simulink model "twozonevavdemo"  (R2020a)
settings: Solver=FixedStepAuto  StartTime=0  StopTime=24*3600  FixedStep=0.1  RelTol=1e-3
PostLoadFcn:
  | if any(exist('dsrtsu_mdlpostloadfcn', 'file') ~= 0), dsrtsu_mdlpostloadfcn('Execute', bdroot); end
InitFcn:
  | , if any(exist('rtifpga_mdlclblib', 'file') ~= 0), rtifpga_mdlclblib('Init', bdroot); end,
  | , if any(exist('dsmpb_private', 'file') ~= 0), dsmpb_private('dsmpb_mdlclblib', 'Init', bdroot); end,
undefined symbols (not defined in the file): dspaceexample_t_dy975j4bckM, newDymolaGui
libraries: dsmpblib x10
PreSaveFcn:
  | , if any(exist('dsmpb_private', 'file') ~= 0), dsmpb_private('dsmpb_mdlclblib', 'PreSave', bdroot); end,
CloseFcn:
  | , if any(exist('dsmpb_private', 'file') ~= 0), dsmpb_private('dsmpb_mdlclblib', 'Close', bdroot); end,
settings Model: RTICANMMDATA=struct('GeneralSetupData',struct('modelroot','D:\github\dspace-modelica-example\simulink\twozonevavdemo','generalsettings',struct('filesettings',struct('destfolder',struct('Name','RTICANMM_FILES','Check',1),'buildfolder',struct('Name','.','Check',1),'AbsDestfolder',struct('Name','D:\github\dspace-modelica-example\simulink\twozonevavdemo\RTICANMM_FILES'),'AbsBuildfolder',struct('Name','D:\github\dspace-modelica-example\simulink\twozonevavdemo'))),'options',struct('addpaths',1,'rmpaths',1,'addtrcexclusion',true,'cannavigator',struct('checkmonitoring',0),'show_usrtrc',0,'use_usrtrc',0),'advanced',struct('options',ones(1,100)),'MPSetup',{{}},'RTI',struct('Type','DSRT','Ver','4.3','Date','02-May-2020'),'modelname','twozonevavdemo','block','twozonevavdemo'))  DSRTSU_INTERNAL_RTIFPGA=160  DSMPB_ID_DATA={'100',struct('BlockId','6dd11bb4-ebec-4f08-8ba6-7ddbcbec7d3b','SignalIds',{{'2fb2bb90-4ec6-48ad-8f81-f1d196760c71'}}),'101',struct('BlockId','2ef807c6-571a-44f3-9a64-946af00fb830','SignalIds',{{'b929fcdd-48af-480b-af6b-b2c3ef490cf9'}}),'102',struct('BlockId','fcb8ffc9-48d0-43e3-97e6-63db34e8a87a','SignalIds',{{'7405cf0b-34b8-4d18-b681-bf257a32f1fc'}}),'103',struct('BlockId','44e3c1f1-df5a-4dd4-b5d4-1957fbd80a33','SignalIds',{{'7449a4d7-6efa-496e-ad1d-0eb127210326'}}),'104',struct('BlockId','d3fc6cbc-e5ea-45da-a1ff-e6d33e572c72','SignalIds',{{'ae88789f-7deb-4ded-bc5a-6d8a92166d0d'}}),'199',struct('BlockId','9376efae-c5ba-4aee-a189-875ca35da0c2','SignalIds',{{'13f0521d-e993-4fe3-8f8d-d5fdd3bf7eee'}}),'200',struct('BlockId','0e030ddc-3f5d-48b0-903c-79a8b3e79f79','SignalIds',{{'2dba2b15-4113-4beb-a147-18d9996277b5'}}),'97',struct('BlockId','c439f065-e928-4c50-b5e3-14eb295499a2','SignalIds',{{'8fe5f31b-da93-4239-8dda-b4cd2b1e3d5b'}}),'98',struct('BlockId','8b35e11d-29bf-41ba-bcb3-e0861426f11f','SignalIds',{{'ce953cd3-6947-465f-be2f-d959c5a96f49'}}),'99',struct('BlockId','4007e34d-3596-41e8-9571-21578a657730','SignalIds',{{'6190f487-0612-4ce8-bb29-664a6f7d7b4d'}})}  Creator=yangyang.fu  LastModifiedBy=yangyang.fu
settings OptimizationCC: BlockReduction=off  ConditionallyExecuteInputs=off  OptimizeBlockIOStorage=off  BufferReuse=off
settings DebuggingCC: TasksWithSamePriorityMsg=none
settings HardwareCC: ProdBitPerPointer=32  ProdBitPerSizeT=32  ProdBitPerPtrDiffT=32  ProdLargestAtomicInteger=Integer  ProdWordSize=32  ProdLongLongMode=on  ProdHWDeviceType=Custom Processor->Custom
settings ModelReferenceCC: EnableParallelModelReferenceBuilds=on
settings SFSimCC: MATLABDynamicMemAlloc=off
settings RTWCC: Description=dSPACE Run-Time Target (for VEOS on Windows and ConfigurationDesk)  SystemTargetFile=dsrt.tlc  GenCodeOnly=on  MakeCommand=make_dsrt  TemplateMakefile=dsrt_default_tmf  RTWVerbose=off  CustomInclude="\"C:\\Program Files\\Dymola 2021\\Source\""
settings STFCustomTargetCC: TargetLangStandard=C99 (ISO)  ParMdlRefBuildCompliant=on  SystemTargetFile=dsrt.tlc
settings GRTTargetCC: CompOptLevelCompliant=off  ConcurrentExecutionCompliant=off  CombineOutputUpdateFcns=off  MatFileLogging=off  CPPClassGenCompliant=off  UseToolchainInfoCompliant=off

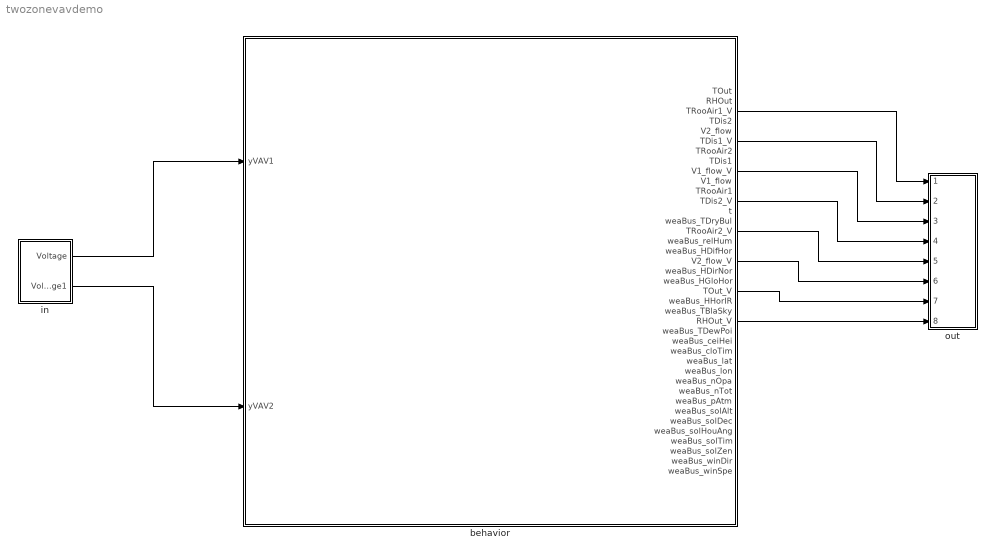
== system twozonevavdemo ==
  behavior : Subsystem
  in : Subsystem
  out : Subsystem
  wires:
  in/1(Voltage) -> behavior/1(yVAV1)
  in/2(Voltage1) -> behavior/2(yVAV2)
  behavior/3(TRooAir1_V) -> out/1(Voltage)
  behavior/6(TDis1_V) -> out/2(Voltage1)
  behavior/9(V1_flow_V) -> out/3(Voltage2)
  behavior/12(TDis2_V) -> out/4(Voltage3)
  behavior/15(TRooAir2_V) -> out/5(Voltage4)
  behavior/18(V2_flow_V) -> out/6(Voltage5)
  behavior/21(TOut_V) -> out/7(Voltage6)
  behavior/24(RHOut_V) -> out/8(Voltage7)

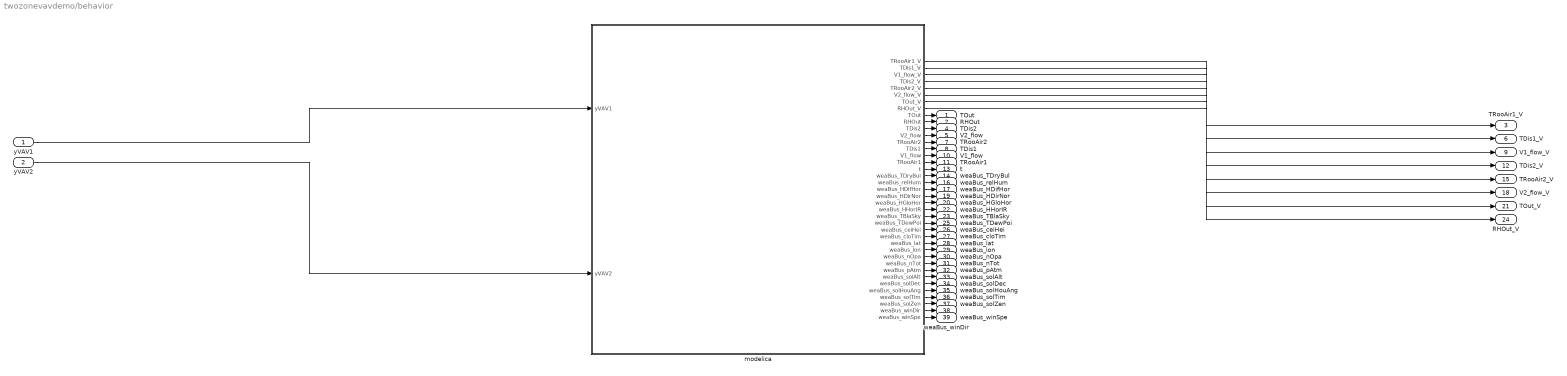
== system twozonevavdemo/behavior ==
  yVAV1 : Inport
  yVAV2 : Inport  Port=2
  modelica : Subsystem  Tag=19-Nov-2021 16:33:56#975  LoadFcn=if exist('newDymolaGui') newDymolaGui('twozonevavdemo/behavior/modelica','PostLoadNew'); else error('Dymola not installed. Must install at least the file newDymolaGui.p'); end;
      mask help:
      | Dymola block.
      | A dymola block allows acausal physical modeling.
      | See Dymola manual for usage.
      settings: CopyFcn=newDymolaGui('19-Nov-2021 16:33:56#975','Copy');  DeleteFcn=if exist('newDymolaGui') newDymolaGui('twozonevavdemo/behavior/modelica','Delete'); end;  NameChangeFcn=newDymolaGui('19-Nov-2021 16:33:56#975','Copy');  OpenFcn=newDymolaGui('twozonevavdemo/behavior/modelica','Init');
      mask Display: image(imread('Dymola.bmp'),[.2,.2,.6,.6])
  TOut : Outport
  RHOut : Outport  Port=2
  TRooAir1_V : Outport  Port=3
  TDis2 : Outport  Port=4
  V2_flow : Outport  Port=5
  TDis1_V : Outport  Port=6
  TRooAir2 : Outport  Port=7
  TDis1 : Outport  Port=8
  V1_flow_V : Outport  Port=9
  V1_flow : Outport  Port=10
  TRooAir1 : Outport  Port=11
  TDis2_V : Outport  Port=12
  t : Outport  Port=13
  weaBus_TDryBul : Outport  Port=14
  TRooAir2_V : Outport  Port=15
  weaBus_relHum : Outport  Port=16
  weaBus_HDifHor : Outport  Port=17
  V2_flow_V : Outport  Port=18
  weaBus_HDirNor : Outport  Port=19
  weaBus_HGloHor : Outport  Port=20
  TOut_V : Outport  Port=21
  weaBus_HHorIR : Outport  Port=22
  weaBus_TBlaSky : Outport  Port=23
  RHOut_V : Outport  Port=24
  weaBus_TDewPoi : Outport  Port=25
  weaBus_ceiHei : Outport  Port=26
  weaBus_cloTim : Outport  Port=27
  weaBus_lat : Outport  Port=28
  weaBus_lon : Outport  Port=29
  weaBus_nOpa : Outport  Port=30
  weaBus_nTot : Outport  Port=31
  weaBus_pAtm : Outport  Port=32
  weaBus_solAlt : Outport  Port=33
  weaBus_solDec : Outport  Port=34
  weaBus_solHouAng : Outport  Port=35
  weaBus_solTim : Outport  Port=36
  weaBus_solZen : Outport  Port=37
  weaBus_winDir : Outport  Port=38
  weaBus_winSpe : Outport  Port=39
  wires:
  yVAV2/1 -> modelica/2(yVAV2)
  modelica/10(RHOut) -> RHOut/1
  modelica/6(V2_flow_V) -> V2_flow_V/1
  modelica/22(weaBus_HGloHor) -> weaBus_HGloHor/1
  modelica/39(weaBus_winSpe) -> weaBus_winSpe/1
  modelica/19(weaBus_relHum) -> weaBus_relHum/1
  modelica/28(weaBus_lat) -> weaBus_lat/1
  yVAV1/1 -> modelica/1(yVAV1)
  modelica/34(weaBus_solDec) -> weaBus_solDec/1
  modelica/7(TOut_V) -> TOut_V/1
  modelica/36(weaBus_solTim) -> weaBus_solTim/1
  modelica/1(TRooAir1_V) -> TRooAir1_V/1
  modelica/3(V1_flow_V) -> V1_flow_V/1
  modelica/16(TRooAir1) -> TRooAir1/1
  modelica/33(weaBus_solAlt) -> weaBus_solAlt/1
  modelica/30(weaBus_nOpa) -> weaBus_nOpa/1
  modelica/2(TDis1_V) -> TDis1_V/1
  modelica/4(TDis2_V) -> TDis2_V/1
  modelica/5(TRooAir2_V) -> TRooAir2_V/1
  modelica/8(RHOut_V) -> RHOut_V/1
  modelica/17(t) -> t/1
  modelica/21(weaBus_HDirNor) -> weaBus_HDirNor/1
  modelica/29(weaBus_lon) -> weaBus_lon/1
  modelica/32(weaBus_pAtm) -> weaBus_pAtm/1
  modelica/35(weaBus_solHouAng) -> weaBus_solHouAng/1
  modelica/38(weaBus_winDir) -> weaBus_winDir/1
  modelica/31(weaBus_nTot) -> weaBus_nTot/1
  modelica/9(TOut) -> TOut/1
  modelica/14(TDis1) -> TDis1/1
  modelica/11(TDis2) -> TDis2/1
  modelica/12(V2_flow) -> V2_flow/1
  modelica/15(V1_flow) -> V1_flow/1
  modelica/23(weaBus_HHorIR) -> weaBus_HHorIR/1
  modelica/20(weaBus_HDifHor) -> weaBus_HDifHor/1
  modelica/18(weaBus_TDryBul) -> weaBus_TDryBul/1
  modelica/13(TRooAir2) -> TRooAir2/1
  modelica/24(weaBus_TBlaSky) -> weaBus_TBlaSky/1
  modelica/26(weaBus_ceiHei) -> weaBus_ceiHei/1
  modelica/27(weaBus_cloTim) -> weaBus_cloTim/1
  modelica/25(weaBus_TDewPoi) -> weaBus_TDewPoi/1
  modelica/37(weaBus_solZen) -> weaBus_solZen/1

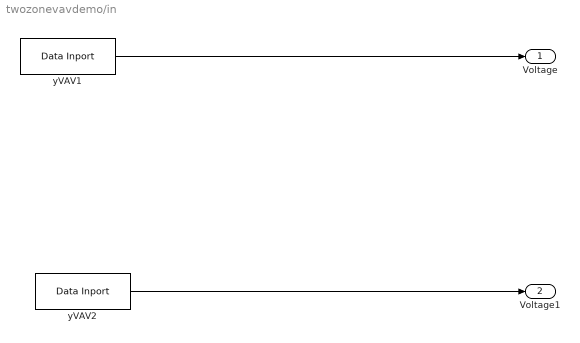
== system twozonevavdemo/in ==
  yVAV1 : dsmpblib/Data Inport  Priority=10000
      settings: SourceProductName=dSPACE Model Interface Blockset
  yVAV2 : dsmpblib/Data Inport  Priority=10000
      settings: SourceProductName=dSPACE Model Interface Blockset
  Voltage : Outport
  Voltage1 : Outport  Port=2
  wires:
  yVAV1/1 -> Voltage/1
  yVAV2/1 -> Voltage1/1

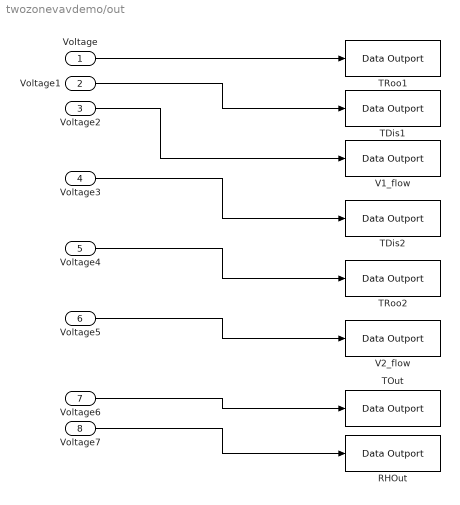
== system twozonevavdemo/out ==
  Voltage : Inport
  Voltage1 : Inport  Port=2
  Voltage2 : Inport  Port=3
  Voltage3 : Inport  Port=4
  Voltage4 : Inport  Port=5
  Voltage5 : Inport  Port=6
  Voltage6 : Inport  Port=7
  Voltage7 : Inport  Port=8
  RHOut : dsmpblib/Data Outport  Priority=-10000
      settings: SourceProductName=dSPACE Model Interface Blockset
  TDis1 : dsmpblib/Data Outport  Priority=-10000
      settings: SourceProductName=dSPACE Model Interface Blockset
  TDis2 : dsmpblib/Data Outport  Priority=-10000
      settings: SourceProductName=dSPACE Model Interface Blockset
  TOut : dsmpblib/Data Outport  Priority=-10000
      settings: SourceProductName=dSPACE Model Interface Blockset
  TRoo1 : dsmpblib/Data Outport  Priority=-10000
      settings: SourceProductName=dSPACE Model Interface Blockset
  TRoo2 : dsmpblib/Data Outport  Priority=-10000
      settings: SourceProductName=dSPACE Model Interface Blockset
  V1_flow : dsmpblib/Data Outport  Priority=-10000
      settings: SourceProductName=dSPACE Model Interface Blockset
  V2_flow : dsmpblib/Data Outport  Priority=-10000
      settings: SourceProductName=dSPACE Model Interface Blockset
  wires:
  Voltage3/1 -> TDis2/1
  Voltage/1 -> TRoo1/1
  Voltage4/1 -> TRoo2/1
  Voltage5/1 -> V2_flow/1
  Voltage7/1 -> RHOut/1
  Voltage2/1 -> V1_flow/1
  Voltage6/1 -> TOut/1
  Voltage1/1 -> TDis1/1

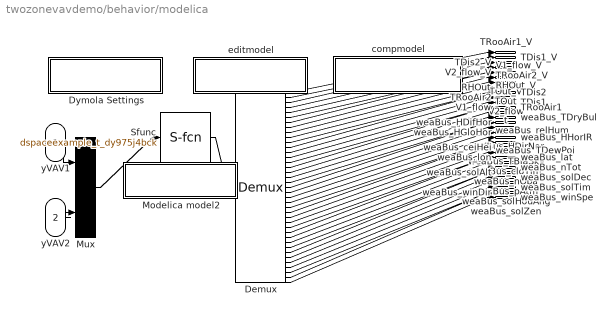
== system twozonevavdemo/behavior/modelica ==
  yVAV1 : Inport
  yVAV2 : Inport  Port=2
  Demux : Demux  Outputs=[1;1;1;1;1;1;1;1;1;1;1;1;1;1;1;1;1;1;1;1;1;1;1;1;1;1;1;1;1;1;1;1;1;1;1;1;1;1;1]
  Dymola Settings : Subsystem  mask{ModelName=dSpaceExample.TwoZoneVAVUnitConverted, MoFileName=D:/github/dspace-modelica-example/dSpaceExample/TwoZoneVAVUnitConverted.mo, dSpace=, BusConnector=[], ResultFile=[], ResultFileOnline=[], ResultDt=[], Libs=:, bigobj=[], ImportFolder=[], guimode=[], ModelName2=[], forRuntime=[], MEXLoad=[], omitDescription=[], ResultName=dspaceexample_t_dy975j4bck}
      mask prompts: ModelName "Name of Dymola model"; MoFileName "File Name (including .mo)"; ResultFile "Create Result"; ResultFileOnline "Load result"; ResultDt "Result min dt"; Libs "Used Libraries"; bigobj "Compiler flag /bigobj"; ImportFolder "Import folder"; guimode "GUI mode flag"; ModelName2 "Model name for import mode"; forRuntime "Runtime export"; MEXLoad "Compiled S-function"; omitDescription "Omit description strings"; ResultName "Name of result file"
      mask Display: disp('Dymola Settings');
  Modelica model2 : Subsystem
      mask Display: disp('Change parameters');
  Mux : Mux  Inputs=[1;1]
  Sfunc : S-Function  Tag=975j4bck  FunctionName=dspaceexample_t_dy975j4bck  Parameters=[dspaceexample_t_dy975j4bckM.pV],[dspaceexample_t_dy975j4bckM.x0V]  PortCounts=[1;1]  SFunctionDeploymentMode=off  EnableBusSupport=off
      mask Display: image(imread('Dymola.bmp'))
  compmodel : Subsystem  InitFcn=newDymolaGui('twozonevavdemo/behavior/modelica','Verify');
      settings: OpenFcn=compileModelica('twozonevavdemo/behavior/modelica');
      mask Display: disp('Compile Modelica model');
  editmodel : Subsystem
      settings: OpenFcn=editModelica('twozonevavdemo/behavior/modelica');
      mask Display: disp('Edit Modelica model');
  TRooAir1_V : Outport
  TDis1_V : Outport  Port=2
  V1_flow_V : Outport  Port=3
  TDis2_V : Outport  Port=4
  TRooAir2_V : Outport  Port=5
  V2_flow_V : Outport  Port=6
  TOut_V : Outport  Port=7
  RHOut_V : Outport  Port=8
  TOut : Outport  Port=9
  RHOut : Outport  Port=10
  TDis2 : Outport  Port=11
  V2_flow : Outport  Port=12
  TRooAir2 : Outport  Port=13
  TDis1 : Outport  Port=14
  V1_flow : Outport  Port=15
  TRooAir1 : Outport  Port=16
  t : Outport  Port=17
  weaBus_TDryBul : Outport  Port=18
  weaBus_relHum : Outport  Port=19
  weaBus_HDifHor : Outport  Port=20
  weaBus_HDirNor : Outport  Port=21
  weaBus_HGloHor : Outport  Port=22
  weaBus_HHorIR : Outport  Port=23
  weaBus_TBlaSky : Outport  Port=24
  weaBus_TDewPoi : Outport  Port=25
  weaBus_ceiHei : Outport  Port=26
  weaBus_cloTim : Outport  Port=27
  weaBus_lat : Outport  Port=28
  weaBus_lon : Outport  Port=29
  weaBus_nOpa : Outport  Port=30
  weaBus_nTot : Outport  Port=31
  weaBus_pAtm : Outport  Port=32
  weaBus_solAlt : Outport  Port=33
  weaBus_solDec : Outport  Port=34
  weaBus_solHouAng : Outport  Port=35
  weaBus_solTim : Outport  Port=36
  weaBus_solZen : Outport  Port=37
  weaBus_winDir : Outport  Port=38
  weaBus_winSpe : Outport  Port=39
  wires:
  Sfunc/1 -> Demux/1
  Demux/1 -> TRooAir1_V/1
  Demux/2 -> TDis1_V/1
  Demux/3 -> V1_flow_V/1
  Demux/4 -> TDis2_V/1
  Demux/5 -> TRooAir2_V/1
  Demux/6 -> V2_flow_V/1
  Demux/7 -> TOut_V/1
  Demux/8 -> RHOut_V/1
  Demux/9 -> TOut/1
  Demux/10 -> RHOut/1
  Demux/11 -> TDis2/1
  Demux/12 -> V2_flow/1
  Demux/13 -> TRooAir2/1
  Demux/14 -> TDis1/1
  Demux/15 -> V1_flow/1
  Demux/16 -> TRooAir1/1
  Demux/17 -> t/1
  Demux/18 -> weaBus_TDryBul/1
  Demux/19 -> weaBus_relHum/1
  Demux/20 -> weaBus_HDifHor/1
  Demux/21 -> weaBus_HDirNor/1
  Demux/22 -> weaBus_HGloHor/1
  Demux/23 -> weaBus_HHorIR/1
  Demux/24 -> weaBus_TBlaSky/1
  Demux/25 -> weaBus_TDewPoi/1
  Demux/26 -> weaBus_ceiHei/1
  Demux/27 -> weaBus_cloTim/1
  Demux/28 -> weaBus_lat/1
  Demux/29 -> weaBus_lon/1
  Demux/30 -> weaBus_nOpa/1
  Demux/31 -> weaBus_nTot/1
  Demux/32 -> weaBus_pAtm/1
  Demux/33 -> weaBus_solAlt/1
  Demux/34 -> weaBus_solDec/1
  Demux/35 -> weaBus_solHouAng/1
  Demux/36 -> weaBus_solTim/1
  Demux/37 -> weaBus_solZen/1
  Demux/38 -> weaBus_winDir/1
  Demux/39 -> weaBus_winSpe/1
  Mux/1 -> Sfunc/1
  yVAV1/1 -> Mux/1
  yVAV2/1 -> Mux/2

== system twozonevavdemo/behavior/modelica/Dymola Settings ==

== system twozonevavdemo/behavior/modelica/Modelica model2 ==

== system twozonevavdemo/behavior/modelica/compmodel ==

== system twozonevavdemo/behavior/modelica/editmodel ==
